simulink model "mIkinBlock"  (R2021a)
settings: Solver=FixedStepAuto  StartTime=0.0  StopTime=20  RelTol=1e-3  EnableMultiTasking=on
libraries: aerolibanimutils x1
settings Model: SILPILModeSetting=veronly  ExtModeTrigDuration=2  Creator=angelo  LastModifiedBy=angelo
settings OptimizationCC: EnhancedBackFolding=on  PassReuseOutputArgsAs=Individual arguments  ZeroExternalMemoryAtStartup=off  ZeroInternalMemoryAtStartup=off  MaxStackSize=64  OptimizeBlockOrder=speed  DifferentSizesBufferReuse=on  OptimizationCustomize=off  EfficientTunableParamExpr=on
settings DebuggingCC: ParameterTunabilityLossMsg=error
settings HardwareCC: ProdBitPerInt=16  ProdBitPerPointer=16  ProdBitPerSizeT=16  ProdBitPerPtrDiffT=16  ProdLargestAtomicFloat=None  ProdWordSize=8  ProdHWDeviceType=Atmel->AVR
settings SFSimCC: MATLABDynamicMemAlloc=off
settings RTWCC: SystemTargetFile=ert.tlc  HardwareBoard=Arduino Mega 2560  TemplateMakefile=ert_default_tmf  Toolchain=Arduino AVR  BuildConfiguration=Faster Runs
settings CodeAppCC: ForceParamTrailComments=on  IgnoreCustomStorageClasses=off  OperatorAnnotations=on  SimulinkDataObjDesc=on  SFDataObjDesc=on  InsertBlockDesc=on
settings ERTTargetCC: SupportContinuousTime=on  SupportVariableSizeSignals=on  ExtModeStaticAllocSize=2048

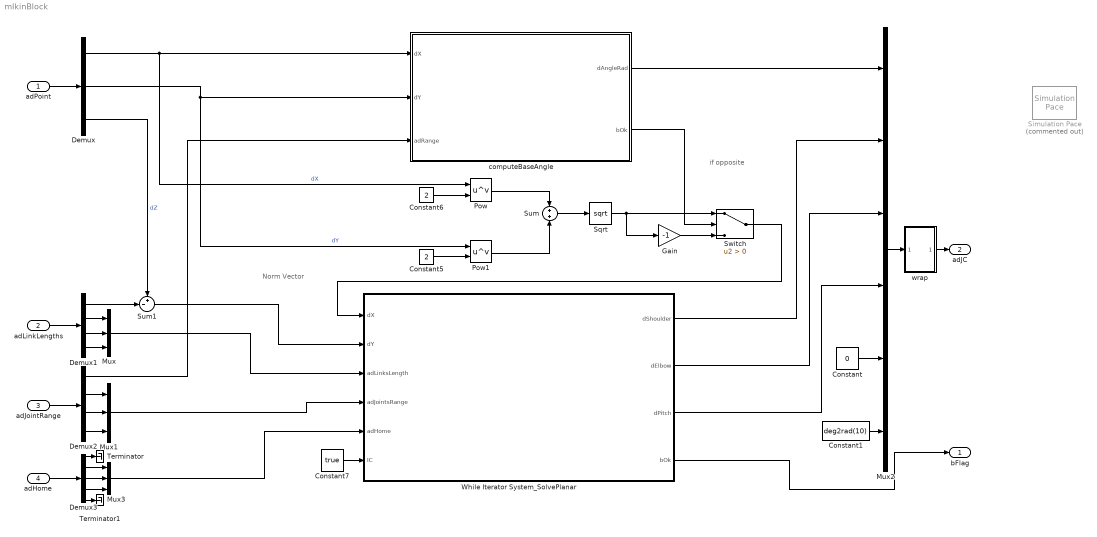
== system mIkinBlock ==
  note: if opposite
  note: Norm Vector
  adPoint : Inport  PortDimensions=3
  adLinkLengths : Inport  Port=2  PortDimensions=4
  adJointRange : Inport  Port=3  PortDimensions=8
  adHome : Inport  Port=4  PortDimensions=5
  Constant : Constant  Value=0
  Constant1 : Constant  Value=deg2rad(10)
  Constant5 : Constant  Value=2
  Constant6 : Constant  Value=2
  Constant7 : Constant  Value=true
  Demux : Demux  Outputs=3
  Demux1 : Demux
  Demux2 : Demux
  Demux3 : Demux  Outputs=5
  Gain : Gain  Gain=-1
  Mux : Mux  Inputs=3
  Mux1 : Mux  Inputs=3
  Mux2 : Mux  Inputs=6
  Mux3 : Mux  Inputs=3
  Pow : Math  Operator=pow  RndMeth=Zero  SaturateOnIntegerOverflow=on
  Pow1 : Math  Operator=pow  RndMeth=Zero  SaturateOnIntegerOverflow=on
  Simulation Pace : aerolibanimutils/Simulation Pace  Commented=on  SimulationPace=1  SleepMode=Auto  OutputPaceError=off  SampleTime=1/30
  Sqrt : Sqrt  SaturateOnIntegerOverflow=on
  Sum : Sum  Inputs=+|+
  Sum1 : Sum  Inputs=+-|
  Switch : Switch  Criteria=u2 > Threshold
  Terminator : Terminator
  Terminator1 : Terminator
  While Iterator System_SolvePlanar : Subsystem  TreatAsAtomicUnit=on
  computeBaseAngle : Subsystem
  wrap : Subsystem
  bFlag : Outport
  adJC : Outport  Port=2  PortDimensions=6
  wires:
  computeBaseAngle/1(dAngleRad) -> Mux2/1
  computeBaseAngle/2(bOk) -> Switch/2
  adPoint/1 -> Demux/1
  Constant6/1 -> Pow/2
  Pow/1 -> Sum/1
  Demux/2 -> Pow1/1, computeBaseAngle/2(dY)  "dY"
  Constant5/1 -> Pow1/2
  Pow1/1 -> Sum/2
  Gain/1 -> Switch/3
  Demux1/1 -> Sum1/2
  Sum/1 -> Sqrt/1
  Sqrt/1 -> Gain/1, Switch/1
  While Iterator System_SolvePlanar/1(dShoulder) -> Mux2/2
  While Iterator System_SolvePlanar/2(dElbow) -> Mux2/3
  While Iterator System_SolvePlanar/3(dPitch) -> Mux2/4
  While Iterator System_SolvePlanar/4(bOk) -> bFlag/1
  Switch/1 -> While Iterator System_SolvePlanar/1(dX)
  Sum1/1 -> While Iterator System_SolvePlanar/2(dY)
  Mux1/1 -> While Iterator System_SolvePlanar/4(adJointsRange)
  Constant7/1 -> While Iterator System_SolvePlanar/6(IC)
  adLinkLengths/1 -> Demux1/1
  Demux1/3 -> Mux/2
  Demux1/2 -> Mux/1
  Demux1/4 -> Mux/3
  Mux/1 -> While Iterator System_SolvePlanar/3(adLinksLength)
  Demux/1 -> Pow/1, computeBaseAngle/1(dX)  "dX"
  Demux/3 -> Sum1/1  "dZ"
  adJointRange/1 -> Demux2/1
  Demux2/4 -> Mux1/3
  Demux2/3 -> Mux1/2
  Demux2/2 -> Mux1/1
  Demux2/1 -> computeBaseAngle/3(adRange)
  Constant/1 -> Mux2/5
  Constant1/1 -> Mux2/6
  Mux2/1 -> wrap/1(In1)
  wrap/1(Out1) -> adJC/1
  Demux3/4 -> Mux3/3
  Demux3/3 -> Mux3/2
  Demux3/1 -> Terminator/1
  Demux3/2 -> Mux3/1
  Demux3/5 -> Terminator1/1
  adHome/1 -> Demux3/1
  Mux3/1 -> While Iterator System_SolvePlanar/5(adHome)

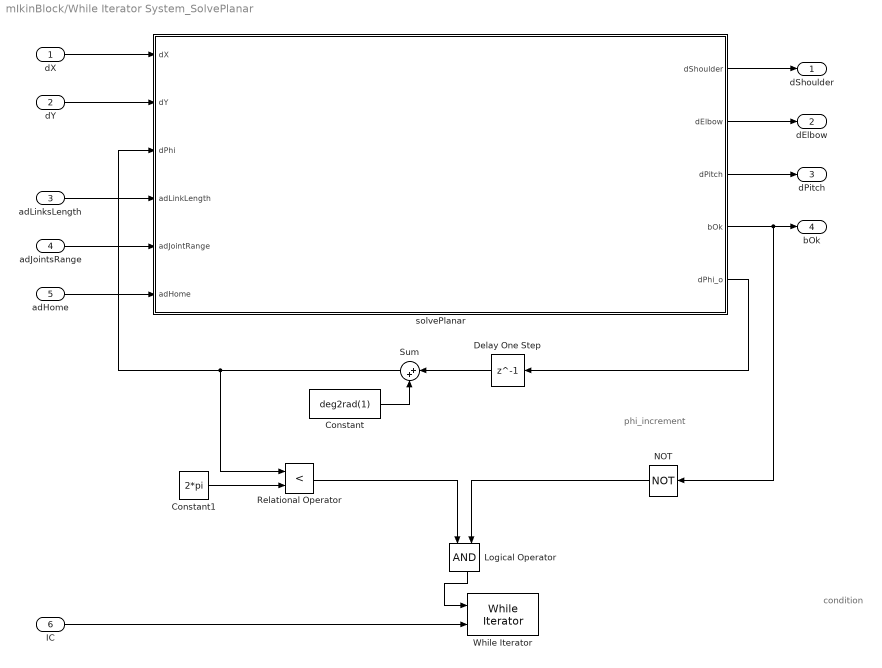
== system mIkinBlock/While Iterator System_SolvePlanar ==
  note: phi_increment
  note: condition
  dX : Inport
  dY : Inport  Port=2
  adLinksLength : Inport  Port=3
  adJointsRange : Inport  Port=4
  adHome : Inport  Port=5
  IC : Inport  Port=6
  Constant : Constant  Value=deg2rad(1)
  Constant1 : Constant  Value=2*pi
  Delay One Step : Delay  DelayLength=1  InitialCondition=deg2rad(-360)
  Logical Operator : Logic  AllPortsSameDT=off  OutDataTypeStr=boolean
  NOT : Logic  Operator=NOT  IconShape=distinctive  AllPortsSameDT=off  OutDataTypeStr=boolean
  Relational Operator : RelationalOperator  Operator=<  OutDataTypeStr=boolean  RndMeth=Simplest
  Sum : Sum  Inputs=|++
  While Iterator : WhileIterator  MaxIters=720  ResetStates=reset
  solvePlanar : Subsystem
  dShoulder : Outport
  dElbow : Outport  Port=2
  dPitch : Outport  Port=3
  bOk : Outport  Port=4
  wires:
  IC/1 -> While Iterator/2
  solvePlanar/1(dShoulder) -> dShoulder/1
  solvePlanar/2(dElbow) -> dElbow/1
  solvePlanar/3(dPitch) -> dPitch/1
  solvePlanar/4(bOk) -> bOk/1, NOT/1
  dX/1 -> solvePlanar/1(dX)
  dY/1 -> solvePlanar/2(dY)
  adLinksLength/1 -> solvePlanar/4(adLinkLength)
  adJointsRange/1 -> solvePlanar/5(adJointRange)
  adHome/1 -> solvePlanar/6(adHome)
  Constant1/1 -> Relational Operator/2
  Relational Operator/1 -> Logical Operator/1
  NOT/1 -> Logical Operator/2
  Logical Operator/1 -> While Iterator/1
  solvePlanar/5(dPhi_o) -> Delay One Step/1
  Delay One Step/1 -> Sum/1
  Sum/1 -> solvePlanar/3(dPhi), Relational Operator/1
  Constant/1 -> Sum/2

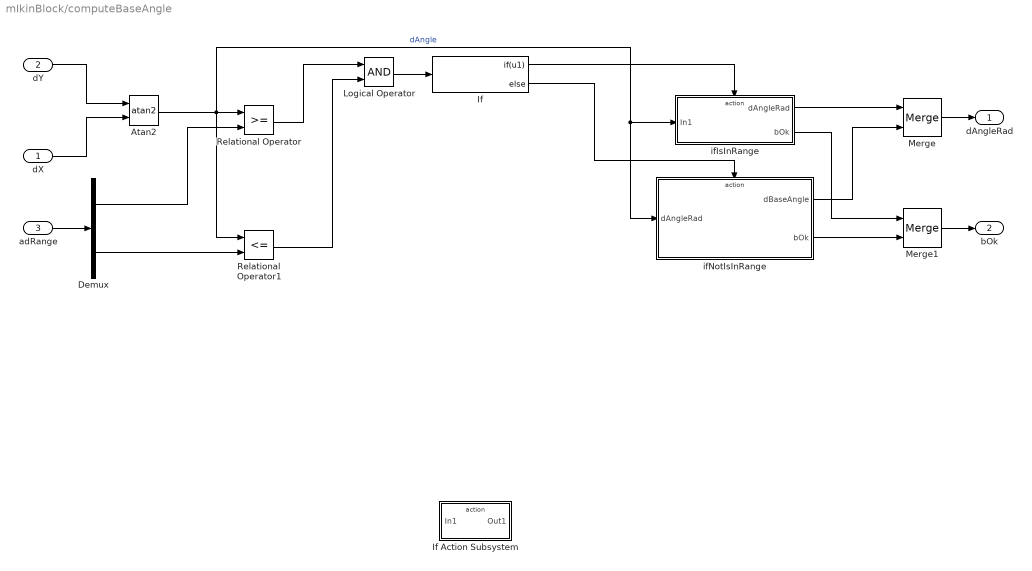
== system mIkinBlock/computeBaseAngle ==
  dX : Inport
  dY : Inport  Port=2
  adRange : Inport  Port=3
  Atan2 : Trigonometry  Operator=atan2
  Demux : Demux  Outputs=2
  If : If  IfExpression=u1
  If Action Subsystem : Subsystem  TreatAsAtomicUnit=on
  Logical Operator : Logic  AllPortsSameDT=off  OutDataTypeStr=boolean
  Merge : Merge
  Merge1 : Merge
  Relational Operator : RelationalOperator  OutDataTypeStr=boolean  RndMeth=Simplest
  Relational Operator1 : RelationalOperator  Operator=<=  OutDataTypeStr=boolean  RndMeth=Simplest
  ifIsInRange : Subsystem  TreatAsAtomicUnit=on
  ifNotIsInRange : Subsystem  TreatAsAtomicUnit=on
  dAngleRad : Outport
  bOk : Outport  Port=2
  wires:
  dX/1 -> Atan2/2
  dY/1 -> Atan2/1
  adRange/1 -> Demux/1
  Atan2/1 -> ifNotIsInRange/1(dAngleRad), ifIsInRange/1(In1), Relational Operator/1, Relational Operator1/1  "dAngle"
  Demux/2 -> Relational Operator1/2
  Demux/1 -> Relational Operator/2
  Relational Operator/1 -> Logical Operator/1
  Relational Operator1/1 -> Logical Operator/2
  Logical Operator/1 -> If/1
  If/1 -> ifIsInRange/Action
  Merge/1 -> dAngleRad/1
  Merge1/1 -> bOk/1
  ifIsInRange/1(dAngleRad) -> Merge/1
  ifIsInRange/2(bOk) -> Merge1/1
  If/2 -> ifNotIsInRange/Action
  ifNotIsInRange/1(dBaseAngle) -> Merge/2
  ifNotIsInRange/2(bOk) -> Merge1/2

== system mIkinBlock/wrap ==
  In1 : Inport
  Constant : Constant  Value=pi/2
  Demux : Demux  Outputs=6
  Mux : Mux  Inputs=3
  Mux1 : Mux
  Sum : Sum  Inputs=|++
  Out1 : Outport
  wires:
  Demux/2 -> Mux1/2
  Demux/5 -> Mux/2
  Constant/1 -> Sum/2
  Demux/3 -> Mux1/3
  Demux/1 -> Mux1/1
  In1/1 -> Demux/1
  Mux/1 -> Out1/1
  Mux1/1 -> Sum/1
  Demux/6 -> Mux/3
  Sum/1 -> Mux/1
  Demux/4 -> Mux1/4

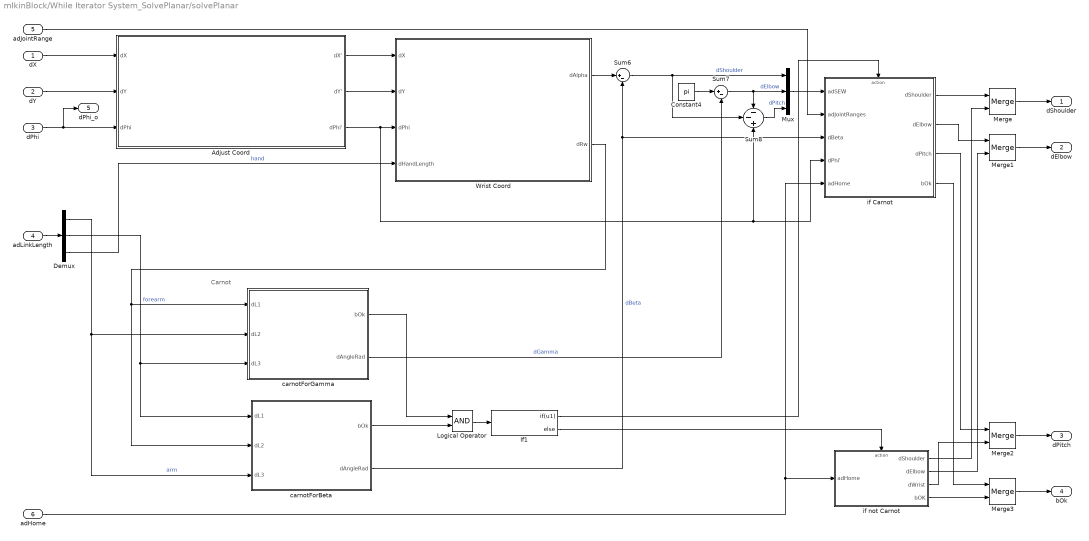
== system mIkinBlock/While Iterator System_SolvePlanar/solvePlanar ==
  note: Carnot
  dX : Inport
  dY : Inport  Port=2
  dPhi : Inport  Port=3
  adLinkLength : Inport  Port=4
  adJointRange : Inport  Port=5
  adHome : Inport  Port=6
  Adjust Coord : Subsystem
  Constant4 : Constant  Value=pi
  Demux : Demux  Outputs=3
  If1 : If  IfExpression=u1
  Logical Operator : Logic  AllPortsSameDT=off  OutDataTypeStr=boolean
  Merge{,1..3} (4 alike) : Merge
  Mux : Mux  Inputs=3
  Sum6 : Sum  Inputs=|+-
  Sum7 : Sum  Inputs=|+-
  Sum8 : Sum  Inputs=--+
  Wrist Coord : Subsystem
  carnotForBeta : MATLAB Function  TreatAsAtomicUnit=on
  carnotForGamma : MATLAB Function  TreatAsAtomicUnit=on
  if Carnot : Subsystem  TreatAsAtomicUnit=on
  if not Carnot : Subsystem  TreatAsAtomicUnit=on
  dShoulder : Outport
  dElbow : Outport  Port=2
  dPitch : Outport  Port=3
  bOk : Outport  Port=4
  dPhi_o : Outport  Port=5
  wires:
  adLinkLength/1 -> Demux/1
  Demux/1 -> carnotForBeta/3(dL3), carnotForGamma/2(dL2)  "arm"
  Demux/2 -> carnotForBeta/1(dL1), carnotForGamma/3(dL3)  "forearm"
  adJointRange/1 -> if Carnot/2(adJointRanges)
  carnotForGamma/2(dAngleRad) -> Sum7/2  "dGamma"
  carnotForBeta/2(dAngleRad) -> Sum6/2, if Carnot/3(dBeta)  "dBeta"
  carnotForGamma/1(bOk) -> Logical Operator/1
  carnotForBeta/1(bOk) -> Logical Operator/2
  Constant4/1 -> Sum7/1
  Adjust Coord/3(dPhi') -> Wrist Coord/3(dPhi), if Carnot/4(dPhi'), Sum8/3
  dX/1 -> Adjust Coord/1(dX)
  dY/1 -> Adjust Coord/2(dY)
  dPhi/1 -> Adjust Coord/3(dPhi), dPhi_o/1
  Wrist Coord/2(dRw) -> carnotForBeta/2(dL2), carnotForGamma/1(dL1)
  Adjust Coord/1(dX') -> Wrist Coord/1(dX)
  Adjust Coord/2(dY') -> Wrist Coord/2(dY)
  Demux/3 -> Wrist Coord/4(dHandLength)  "hand"
  Sum6/1 -> Mux/1, Sum8/2  "dShoulder"
  Sum7/1 -> Sum8/1, Mux/2  "dElbow"
  Sum8/1 -> Mux/3  "dPitch"
  Merge/1 -> dShoulder/1
  Merge1/1 -> dElbow/1
  Merge2/1 -> dPitch/1
  Merge3/1 -> bOk/1
  Logical Operator/1 -> If1/1
  If1/1 -> if Carnot/Action
  If1/2 -> if not Carnot/Action
  adHome/1 -> if Carnot/5(adHome), if not Carnot/1(adHome)
  Mux/1 -> if Carnot/1(adSEW)
  if Carnot/1(dShoulder) -> Merge/1
  if Carnot/2(dElbow) -> Merge1/1
  if Carnot/3(dPitch) -> Merge2/1
  if Carnot/4(bOk) -> Merge3/1
  if not Carnot/4(bOK) -> Merge3/2
  if not Carnot/1(dShoulder) -> Merge/2
  if not Carnot/2(dElbow) -> Merge1/2
  if not Carnot/3(dWrist) -> Merge2/2
  Wrist Coord/1(dAlpha) -> Sum6/1

== system mIkinBlock/computeBaseAngle/If Action Subsystem ==
  In1 : Inport
  Action Port : ActionPort
  Out1 : Outport
  wires:
  In1/1 -> Out1/1

== system mIkinBlock/computeBaseAngle/ifIsInRange ==
  In1 : Inport
  Action Port : ActionPort  ActionPortLabel=if(u1)
  Constant : Constant  Value=true
  dAngleRad : Outport
  bOk : Outport  Port=2
  wires:
  In1/1 -> dAngleRad/1
  Constant/1 -> bOk/1

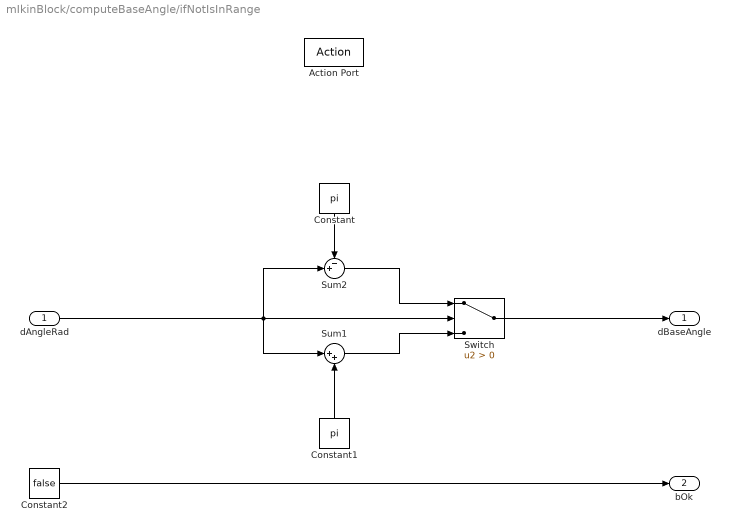
== system mIkinBlock/computeBaseAngle/ifNotIsInRange ==
  dAngleRad : Inport
  Action Port : ActionPort  ActionPortLabel=else
  Constant : Constant  Value=pi
  Constant1 : Constant  Value=pi
  Constant2 : Constant  Value=false
  Sum1 : Sum  Inputs=|++
  Sum2 : Sum  Inputs=-+|
  Switch : Switch  Criteria=u2 > Threshold
  dBaseAngle : Outport
  bOk : Outport  Port=2
  wires:
  dAngleRad/1 -> Sum2/2, Sum1/1, Switch/2
  Constant/1 -> Sum2/1
  Sum2/1 -> Switch/1
  Sum1/1 -> Switch/3
  Constant1/1 -> Sum1/2
  Switch/1 -> dBaseAngle/1
  Constant2/1 -> bOk/1

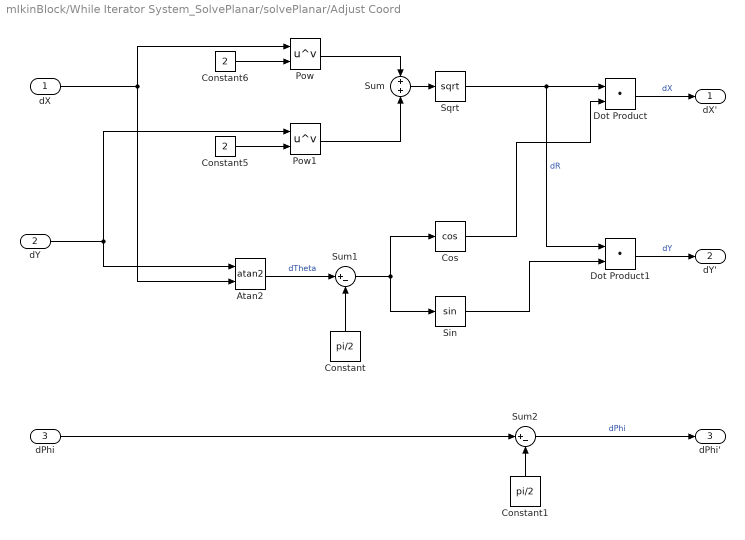
== system mIkinBlock/While Iterator System_SolvePlanar/solvePlanar/Adjust Coord ==
  dX : Inport
  dY : Inport  Port=2
  dPhi : Inport  Port=3
  Atan2 : Trigonometry  Operator=atan2
  Constant : Constant  Value=pi/2
  Constant1 : Constant  Value=pi/2
  Constant5 : Constant  Value=2
  Constant6 : Constant  Value=2
  Cos : Trigonometry  Operator=cos
  Dot Product : DotProduct  InputSameDT=on  OutDataTypeStr=Inherit: Inherit via internal rule
  Dot Product1 : DotProduct  InputSameDT=on  OutDataTypeStr=Inherit: Inherit via internal rule
  Pow : Math  Operator=pow  RndMeth=Zero  SaturateOnIntegerOverflow=on
  Pow1 : Math  Operator=pow  RndMeth=Zero  SaturateOnIntegerOverflow=on
  Sin : Trigonometry
  Sqrt : Sqrt  SaturateOnIntegerOverflow=on
  Sum : Sum  Inputs=+|+
  Sum1 : Sum  Inputs=|+-
  Sum2 : Sum  Inputs=|+-
  dX' : Outport
  dY' : Outport  Port=2
  dPhi' : Outport  Port=3
  wires:
  Constant/1 -> Sum1/2
  Pow1/1 -> Sum/2
  dY/1 -> Pow1/1, Atan2/1
  Sin/1 -> Dot Product1/2
  Sum2/1 -> dPhi'/1  "dPhi"
  Dot Product/1 -> dX'/1  "dX"
  Constant6/1 -> Pow/2
  Dot Product1/1 -> dY'/1  "dY"
  dX/1 -> Pow/1, Atan2/2
  Constant1/1 -> Sum2/2
  Sum1/1 -> Sin/1, Cos/1
  Constant5/1 -> Pow1/2
  Sum/1 -> Sqrt/1
  dPhi/1 -> Sum2/1
  Sqrt/1 -> Dot Product1/1, Dot Product/1  "dR"
  Atan2/1 -> Sum1/1  "dTheta"
  Pow/1 -> Sum/1
  Cos/1 -> Dot Product/2

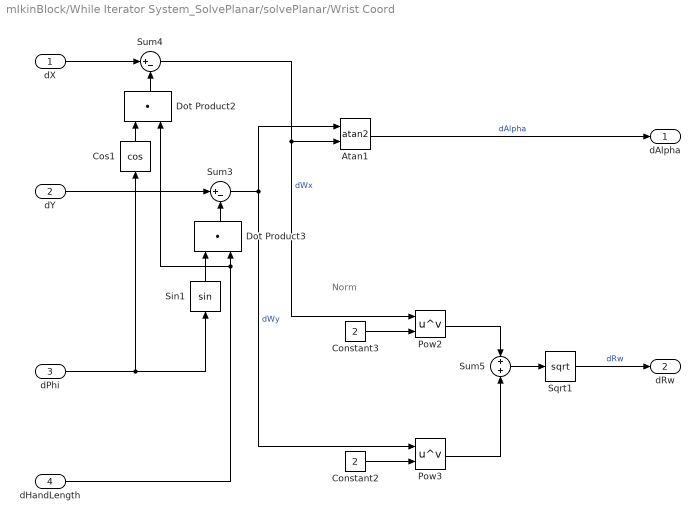
== system mIkinBlock/While Iterator System_SolvePlanar/solvePlanar/Wrist Coord ==
  note: Norm
  dX : Inport
  dY : Inport  Port=2
  dPhi : Inport  Port=3
  dHandLength : Inport  Port=4
  Atan1 : Trigonometry  Operator=atan2
  Constant2 : Constant  Value=2
  Constant3 : Constant  Value=2
  Cos1 : Trigonometry  Operator=cos
  Dot Product2 : DotProduct  InputSameDT=on  OutDataTypeStr=Inherit: Inherit via internal rule
  Dot Product3 : DotProduct  InputSameDT=on  OutDataTypeStr=Inherit: Inherit via internal rule
  Pow2 : Math  Operator=pow  RndMeth=Zero  SaturateOnIntegerOverflow=on
  Pow3 : Math  Operator=pow  RndMeth=Zero  SaturateOnIntegerOverflow=on
  Sin1 : Trigonometry
  Sqrt1 : Sqrt  SaturateOnIntegerOverflow=on
  Sum3 : Sum  Inputs=|+-
  Sum4 : Sum  Inputs=|+-
  Sum5 : Sum  Inputs=+|+
  dAlpha : Outport
  dRw : Outport  Port=2
  wires:
  Constant3/1 -> Pow2/2
  dHandLength/1 -> Dot Product3/2, Dot Product2/2
  Pow2/1 -> Sum5/1
  Sqrt1/1 -> dRw/1  "dRw"
  Pow3/1 -> Sum5/2
  Sum5/1 -> Sqrt1/1
  dPhi/1 -> Sin1/1, Cos1/1
  Atan1/1 -> dAlpha/1  "dAlpha"
  dX/1 -> Sum4/1
  Sum4/1 -> Pow2/1, Atan1/2  "dWx"
  Sin1/1 -> Dot Product3/1
  Dot Product2/1 -> Sum4/2
  Sum3/1 -> Pow3/1, Atan1/1  "dWy"
  Constant2/1 -> Pow3/2
  Dot Product3/1 -> Sum3/2
  dY/1 -> Sum3/1
  Cos1/1 -> Dot Product2/1

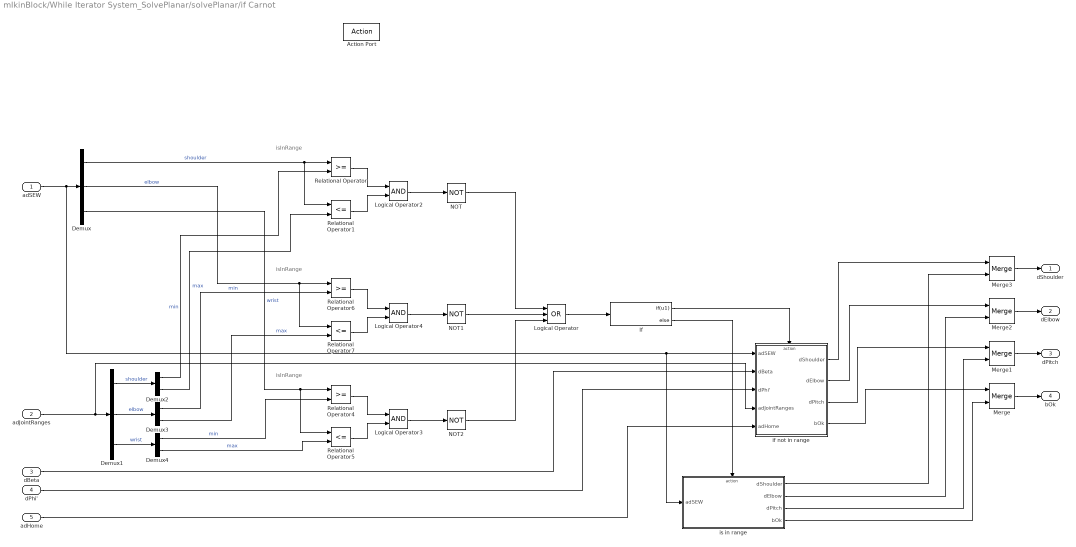
== system mIkinBlock/While Iterator System_SolvePlanar/solvePlanar/if Carnot ==
  note: isInRange
  note: isInRange
  note: isInRange
  adSEW : Inport
  adJointRanges : Inport  Port=2
  dBeta : Inport  Port=3
  dPhi' : Inport  Port=4
  adHome : Inport  Port=5
  Action Port : ActionPort  ActionPortLabel=if(u1)
  Demux : Demux  Outputs=3
  Demux1 : Demux  Outputs=3
  Demux2 : Demux  Outputs=2
  Demux3 : Demux  Outputs=2
  Demux4 : Demux  Outputs=2
  If : If  IfExpression=u1
  Logical Operator : Logic  Operator=OR  Inputs=3  AllPortsSameDT=off  OutDataTypeStr=boolean
  Logical Operator2 : Logic  AllPortsSameDT=off  OutDataTypeStr=boolean
  Logical Operator3 : Logic  AllPortsSameDT=off  OutDataTypeStr=boolean
  Logical Operator4 : Logic  AllPortsSameDT=off  OutDataTypeStr=boolean
  Merge{,1..3} (4 alike) : Merge
  NOT : Logic  Operator=NOT  IconShape=distinctive  AllPortsSameDT=off  OutDataTypeStr=boolean
  NOT1 : Logic  Operator=NOT  IconShape=distinctive  AllPortsSameDT=off  OutDataTypeStr=boolean
  NOT2 : Logic  Operator=NOT  IconShape=distinctive  AllPortsSameDT=off  OutDataTypeStr=boolean
  Relational Operator : RelationalOperator  OutDataTypeStr=boolean  RndMeth=Simplest
  Relational Operator1 : RelationalOperator  Operator=<=  OutDataTypeStr=boolean  RndMeth=Simplest
  Relational Operator4 : RelationalOperator  OutDataTypeStr=boolean  RndMeth=Simplest
  Relational Operator5 : RelationalOperator  Operator=<=  OutDataTypeStr=boolean  RndMeth=Simplest
  Relational Operator6 : RelationalOperator  OutDataTypeStr=boolean  RndMeth=Simplest
  Relational Operator7 : RelationalOperator  Operator=<=  OutDataTypeStr=boolean  RndMeth=Simplest
  if not in range : Subsystem  TreatAsAtomicUnit=on
  is in range : Subsystem  TreatAsAtomicUnit=on
  dShoulder : Outport
  dElbow : Outport  Port=2
  dPitch : Outport  Port=3
  bOk : Outport  Port=4
  wires:
  Demux1/3 -> Demux4/1  "wrist"
  Demux1/2 -> Demux3/1  "elbow"
  Demux3/2 -> Relational Operator7/2  "max"
  Demux2/2 -> Relational Operator1/2  "max"
  Demux3/1 -> Relational Operator6/2  "min"
  Demux2/1 -> Relational Operator/2  "min"
  Demux1/1 -> Demux2/1  "shoulder"
  Demux4/1 -> Relational Operator4/2  "min"
  Demux4/2 -> Relational Operator5/2  "max"
  adJointRanges/1 -> if not in range/4(adJointRanges), Demux1/1
  adSEW/1 -> is in range/1(adSEW), if not in range/1(adSEW), Demux/1
  Demux/1 -> Relational Operator1/1, Relational Operator/1  "shoulder"
  Demux/2 -> Relational Operator7/1, Relational Operator6/1  "elbow"
  Demux/3 -> Relational Operator5/1, Relational Operator4/1  "wrist"
  Relational Operator/1 -> Logical Operator2/1
  Relational Operator1/1 -> Logical Operator2/2
  Relational Operator5/1 -> Logical Operator3/2
  Relational Operator4/1 -> Logical Operator3/1
  Relational Operator6/1 -> Logical Operator4/1
  Relational Operator7/1 -> Logical Operator4/2
  Logical Operator2/1 -> NOT/1
  Logical Operator4/1 -> NOT1/1
  Logical Operator3/1 -> NOT2/1
  NOT/1 -> Logical Operator/1
  NOT1/1 -> Logical Operator/2
  NOT2/1 -> Logical Operator/3
  Logical Operator/1 -> If/1
  If/1 -> if not in range/Action
  If/2 -> is in range/Action
  Merge/1 -> bOk/1
  Merge2/1 -> dElbow/1
  Merge1/1 -> dPitch/1
  Merge3/1 -> dShoulder/1
  if not in range/4(bOk) -> Merge/1
  is in range/4(bOk) -> Merge/2
  if not in range/1(dShoulder) -> Merge3/1
  is in range/1(dShoulder) -> Merge3/2
  if not in range/2(dElbow) -> Merge2/1
  is in range/2(dElbow) -> Merge2/2
  if not in range/3(dPitch) -> Merge1/1
  is in range/3(dPitch) -> Merge1/2
  dBeta/1 -> if not in range/2(dBeta)
  dPhi'/1 -> if not in range/3(dPhi')
  adHome/1 -> if not in range/5(adHome)

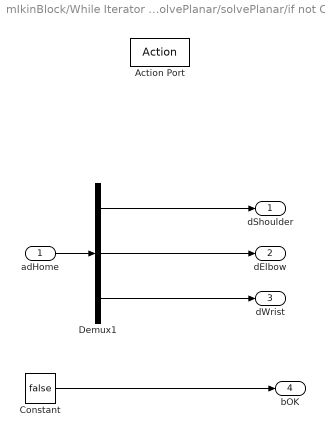
== system mIkinBlock/While Iterator System_SolvePlanar/solvePlanar/if not Carnot ==
  adHome : Inport
  Action Port : ActionPort  ActionPortLabel=else
  Constant : Constant  Value=false
  Demux1 : Demux  Outputs=3
  dShoulder : Outport
  dElbow : Outport  Port=2
  dWrist : Outport  Port=3
  bOK : Outport  Port=4
  wires:
  Constant/1 -> bOK/1
  adHome/1 -> Demux1/1
  Demux1/3 -> dWrist/1
  Demux1/2 -> dElbow/1
  Demux1/1 -> dShoulder/1

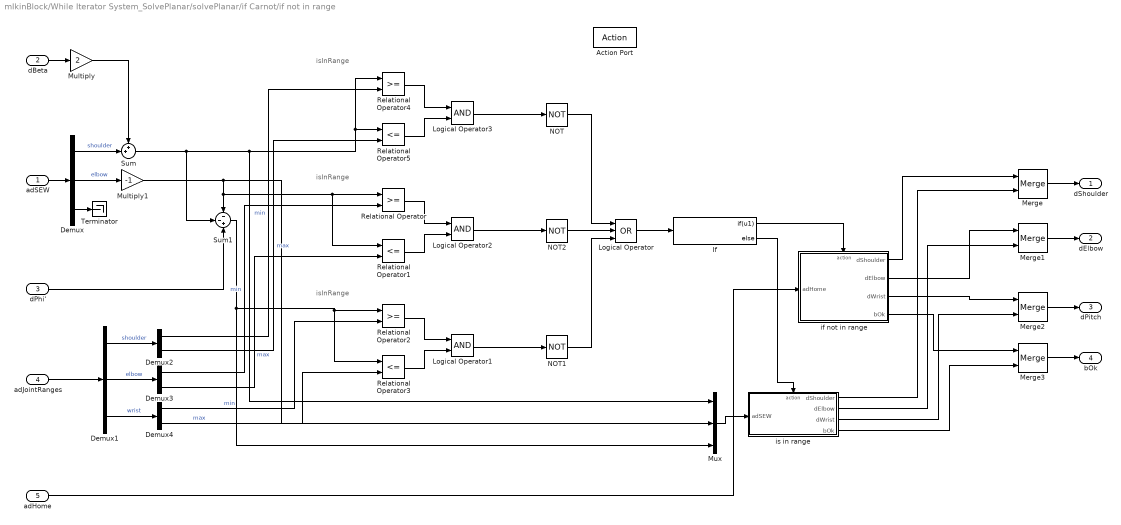
== system mIkinBlock/While Iterator System_SolvePlanar/solvePlanar/if Carnot/if not in range ==
  note: isInRange
  note: isInRange
  note: isInRange
  adSEW : Inport
  dBeta : Inport  Port=2
  dPhi' : Inport  Port=3
  adJointRanges : Inport  Port=4
  adHome : Inport  Port=5
  Action Port : ActionPort  ActionPortLabel=if(u1)
  Demux : Demux  Outputs=3
  Demux1 : Demux  Outputs=3
  Demux2 : Demux  Outputs=2
  Demux3 : Demux  Outputs=2
  Demux4 : Demux  Outputs=2
  If : If  IfExpression=u1
  Logical Operator : Logic  Operator=OR  Inputs=3  AllPortsSameDT=off  OutDataTypeStr=boolean
  Logical Operator1 : Logic  AllPortsSameDT=off  OutDataTypeStr=boolean
  Logical Operator2 : Logic  AllPortsSameDT=off  OutDataTypeStr=boolean
  Logical Operator3 : Logic  AllPortsSameDT=off  OutDataTypeStr=boolean
  Merge{,1..3} (4 alike) : Merge
  Multiply : Gain  Gain=2
  Multiply1 : Gain  Gain=-1
  Mux : Mux  Inputs=3
  NOT : Logic  Operator=NOT  IconShape=distinctive  AllPortsSameDT=off  OutDataTypeStr=boolean
  NOT1 : Logic  Operator=NOT  IconShape=distinctive  AllPortsSameDT=off  OutDataTypeStr=boolean
  NOT2 : Logic  Operator=NOT  IconShape=distinctive  AllPortsSameDT=off  OutDataTypeStr=boolean
  Relational Operator : RelationalOperator  OutDataTypeStr=boolean  RndMeth=Simplest
  Relational Operator1 : RelationalOperator  Operator=<=  OutDataTypeStr=boolean  RndMeth=Simplest
  Relational Operator2 : RelationalOperator  OutDataTypeStr=boolean  RndMeth=Simplest
  Relational Operator3 : RelationalOperator  Operator=<=  OutDataTypeStr=boolean  RndMeth=Simplest
  Relational Operator4 : RelationalOperator  OutDataTypeStr=boolean  RndMeth=Simplest
  Relational Operator5 : RelationalOperator  Operator=<=  OutDataTypeStr=boolean  RndMeth=Simplest
  Sum : Sum  Inputs=++|
  Sum1 : Sum  Inputs=--+
  Terminator : Terminator
  if not in range : Subsystem  TreatAsAtomicUnit=on
  is in range : Subsystem  TreatAsAtomicUnit=on
  dShoulder : Outport
  dElbow : Outport  Port=2
  dPitch : Outport  Port=3
  bOk : Outport  Port=4
  wires:
  adSEW/1 -> Demux/1
  Demux/1 -> Sum/2  "shoulder"
  dBeta/1 -> Multiply/1
  Multiply/1 -> Sum/1
  Demux/2 -> Multiply1/1  "elbow"
  Sum/1 -> Sum1/2, Mux/1, Relational Operator4/1, Relational Operator5/1
  Multiply1/1 -> Mux/2, Relational Operator1/1, Relational Operator/1, Sum1/1
  dPhi'/1 -> Sum1/3
  Demux/3 -> Terminator/1
  Sum1/1 -> Mux/3, Relational Operator3/1, Relational Operator2/1
  Merge/1 -> dShoulder/1
  Merge1/1 -> dElbow/1
  Merge2/1 -> dPitch/1
  Merge3/1 -> bOk/1
  Demux1/3 -> Demux4/1  "wrist"
  Demux1/2 -> Demux3/1  "elbow"
  adJointRanges/1 -> Demux1/1
  Demux1/1 -> Demux2/1  "shoulder"
  Relational Operator1/1 -> Logical Operator2/2
  Relational Operator/1 -> Logical Operator2/1
  Relational Operator2/1 -> Logical Operator1/1
  Relational Operator3/1 -> Logical Operator1/2
  Relational Operator4/1 -> Logical Operator3/1
  Relational Operator5/1 -> Logical Operator3/2
  Demux2/1 -> Relational Operator4/2  "min"
  Demux2/2 -> Relational Operator5/2  "max"
  Demux3/1 -> Relational Operator/2  "min"
  Demux3/2 -> Relational Operator1/2  "max"
  Demux4/1 -> Relational Operator2/2  "min"
  Demux4/2 -> Relational Operator3/2  "max"
  Logical Operator3/1 -> NOT/1
  Logical Operator2/1 -> NOT2/1
  Logical Operator1/1 -> NOT1/1
  NOT2/1 -> Logical Operator/2
  NOT/1 -> Logical Operator/1
  NOT1/1 -> Logical Operator/3
  Logical Operator/1 -> If/1
  If/1 -> if not in range/Action
  If/2 -> is in range/Action
  if not in range/4(bOk) -> Merge3/1
  adHome/1 -> if not in range/1(adHome)
  is in range/4(bOk) -> Merge3/2
  if not in range/3(dWrist) -> Merge2/1
  if not in range/2(dElbow) -> Merge1/1
  if not in range/1(dShoulder) -> Merge/1
  is in range/1(dShoulder) -> Merge/2
  is in range/2(dElbow) -> Merge1/2
  is in range/3(dWrist) -> Merge2/2
  Mux/1 -> is in range/1(adSEW)

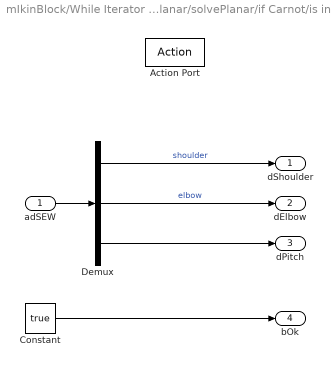
== system mIkinBlock/While Iterator System_SolvePlanar/solvePlanar/if Carnot/is in range ==
  adSEW : Inport
  Action Port : ActionPort  ActionPortLabel=else
  Constant : Constant  Value=true
  Demux : Demux  Outputs=3
  dShoulder : Outport
  dElbow : Outport  Port=2
  dPitch : Outport  Port=3
  bOk : Outport  Port=4
  wires:
  Constant/1 -> bOk/1
  adSEW/1 -> Demux/1
  Demux/1 -> dShoulder/1  "shoulder"
  Demux/2 -> dElbow/1  "elbow"
  Demux/3 -> dPitch/1

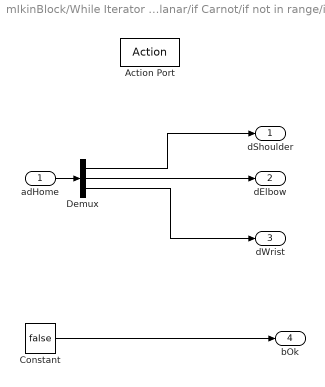
== system mIkinBlock/While Iterator System_SolvePlanar/solvePlanar/if Carnot/if not in range/if not in range ==
  adHome : Inport
  Action Port : ActionPort  ActionPortLabel=if(u1)
  Constant : Constant  Value=false
  Demux : Demux  Outputs=3
  dShoulder : Outport
  dElbow : Outport  Port=2
  dWrist : Outport  Port=3
  bOk : Outport  Port=4
  wires:
  Constant/1 -> bOk/1
  adHome/1 -> Demux/1
  Demux/1 -> dShoulder/1
  Demux/3 -> dWrist/1
  Demux/2 -> dElbow/1

== system mIkinBlock/While Iterator System_SolvePlanar/solvePlanar/if Carnot/if not in range/is in range ==
  adSEW : Inport
  Action Port : ActionPort  ActionPortLabel=else
  Constant : Constant  Value=true
  Demux : Demux  Outputs=3
  dShoulder : Outport
  dElbow : Outport  Port=2
  dWrist : Outport  Port=3
  bOk : Outport  Port=4
  wires:
  Constant/1 -> bOk/1
  adSEW/1 -> Demux/1
  Demux/1 -> dShoulder/1
  Demux/2 -> dElbow/1
  Demux/3 -> dWrist/1

== matlab function mIkinBlock/While Iterator System_SolvePlanar/solvePlanar/carnotForGamma ==
  data: dL1 input; bOk output; dL2 input; dL3 input; dAngleRad output
function [bOk, dAngleRad] = carnotRule(dL1, dL2, dL3)

if (dL1 <= 0 || dL2 <= 0 || dL3 <= 0)
    bOk         = false;
    dAngleRad   = 0.0;
    return;
end

dC23 = (dL2^2 + dL3^2 - dL1^2) / (2* dL2 * dL3);

if (dC23 > 1 || dC23 < -1)
    bOk         = false;
    dAngleRad   = 0.0;
    return;
end

dAngleRad = acos(dC23);
bOk = true;

end

== matlab function mIkinBlock/While Iterator System_SolvePlanar/solvePlanar/carnotForBeta ==
  data: dL1 input; bOk output; dL2 input; dL3 input; dAngleRad output
function [bOk, dAngleRad] = carnotRule(dL1, dL2, dL3)

if (dL1 <= 0 || dL2 <= 0 || dL3 <= 0)
    bOk         = false;
    dAngleRad   = 0.0;
    return;
end

dC23 = (dL2^2 + dL3^2 - dL1^2) / (2* dL2 * dL3);

if (dC23 > 1 || dC23 < -1)
    bOk         = false;
    dAngleRad   = 0.0;
    return;
end

dAngleRad = acos(dC23);
bOk = true;

end
